simulink model "FuzzyNeuro_neuesNetz"  (Simulink 7.8)
settings: Solver=ode1  StartTime=0.0  StopTime=inf  FixedStep=0.01  RelTol=1e-3
PostLoadFcn:
  | , if any(exist('dsrtsu_mdlpostloadfcn', 'file') == [2, 3, 6]), try dsrtsu_mdlpostloadfcn('Execute', bdroot); catch fprintf('Error in PostLoadFcn (dsrtsu_mdlpostloadfcn) for model "%s":\n %s\n', bdroot, lasterr); end, end,
undefined symbols (not defined in the file): Faktorh1, Faktorh2, Faktorh3, Offseth1, Offseth2, Offseth3
libraries: neural x14, rtilib1104 x13, fuzblock x1
CloseFcn:
  | rtwprivate ssgencode ModelCloseRequest FuzzyNeuro
settings Model: DSRTSU_INTERNAL_RTI_VER=390  DSRTSU_INTERNAL_RTI_TYPE=rti1104  Creator=pendel  LastModifiedBy=pendel  ExtModeArmWhenConnect=off  BufferReuse=off
settings OptimizationCC: BlockReduction=off  BooleanDataType=off  OptimizeBlockIOStorage=off  BufferReuse=off  ExpressionFolding=off  LocalBlockOutputs=off  InitFltsAndDblsToZero=on
settings DebuggingCC: SaveWithParameterizedLinksMsg=none  SignalResolutionControl=TryResolveAllWithWarning  SolverPrmCheckMsg=none  MultiTaskDSMMsg=warning  MultiTaskCondExecSysMsg=none  FcnCallInpInsideContextMsg=Use local settings
settings HardwareCC: ProdIntDivRoundTo=Zero  ProdEndianess=BigEndian  ProdHWDeviceType=Generic->Custom  TargetIntDivRoundTo=Zero  TargetEndianess=BigEndian  TargetHWDeviceType=Generic->Custom
settings RTWCC: SystemTargetFile=rti1104.tlc  MakeCommand=make_rti  TemplateMakefile=rti1104.tmf  Description=dSPACE DS1104 Hardware Platform  RTWVerbose=off  RetainRTWFile=on  ProcessScript=rti1104_make_rtw_hook  IncludeERTFirstTime=on
settings CodeAppCC: IncHierarchyInIds=on
settings STFCustomTargetCC: TargetFcnLib=ansi_tfl_tmw.mat  ParMdlRefBuildCompliant=on  SystemTargetFile=rti1104.tlc
settings GRTTargetCC: TargetFcnLib=ansi_tfl_tmw.mat  CompOptLevelCompliant=off  ConcurrentExecutionCompliant=off  MatFileLogging=off  ExtMode=on  ExtModeMexFile=noextcomm
settings CustomProperty: DataType=RTWOptions_EnumType_C__dSPACE RCPHIL 72_matlab_rti1104_tlc_rti1104_1InitialSimState  Value=RUN
settings EnumStrPairs: String=RUN

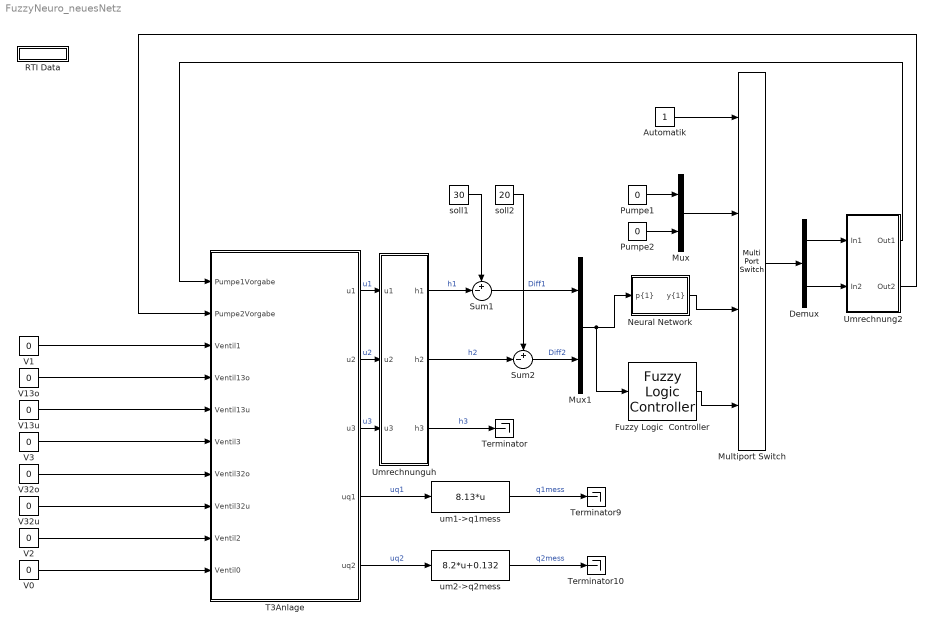
== system FuzzyNeuro_neuesNetz ==
  Automatik : Constant
  Demux : Demux  Outputs=2
  Fuzzy Logic  Controller : fuzblock/Fuzzy Logic  Controller  fis=Schmid
  Multiport Switch : MultiPortSwitch  zeroidx=off  SaturateOnIntegerOverflow=on  InputSameDT=on
  Mux : Mux  Inputs=2
  Mux1 : Mux  Inputs=2
  Neural Network : Subsystem
  Pumpe1 : Constant  Value=0
  Pumpe2 : Constant  Value=0
  RTI Data : Subsystem  Tag=struct('RTIDataServer',struct('RTIDataServerVs','2','RTIModelDescription','struct(''main'',''FuzzyNeuro_neuesNetz'',''sub'','''',''isMp'',0)'))  LoadFcn="if exist('rtidc'), try,  rtidc('DataHostBlockClbLoad', gcbh); catch, disp(['Warning: ''LoadFcn'' for RTI Data block failed: ' lasterr]); end, end,"
      settings: CopyFcn="if exist('rtidc'), try,  rtidc('DataHostBlockClbCopy', gcbh); catch, disp(['Warning: ''CopyFcn'' for RTI Data block failed: ' lasterr]); end, end,"  DeleteFcn="if exist('rtidc'), try,  rtidc('DataHostBlockClbDelete', gcbh); catch, disp(['Warning: ''DeleteFcn'' for RTI Data block failed: ' lasterr]); end, end,"  ModelCloseFcn="if exist('rtidc'), try,  rtidc('DataHostBlockClbModelClose', gcbh); catch, disp(['Warning: ''ModelCloseFcn'' for RTI Data block failed: ' lasterr]); end, end,"  PreSaveFcn="if exist('rtidc'), try,  rtidc('DataHostBlockClbPreSave', gcbh); catch, disp(['Warning: ''PreSaveFcn'' for RTI Data block failed: ' lasterr]); end, end,"  PostSaveFcn="if exist('rtidc'), try,  rtidc('DataHostBlockClbPostSave', gcbh); catch, disp(['Warning: ''PostSaveFcn'' for RTI Data block failed: ' lasterr]); end, end,"  NameChangeFcn="if exist('rtidc'), try,  rtidc('DataHostBlockClbNameChange', gcbh); catch, disp(['Warning: ''NameChangeFcn'' for RTI Data block failed: ' lasterr]); end, end,"
      mask Type: RTI_DATA_HOST
      mask Description:
      | RTI Data Block.
      | This block is used by RTI to store internal model-dependent data.
      | Please keep this block on the root level of the model. Deleting this block will result in data loss.
      | 
      | NEVER DELETE OR COPY THIS BLOCK!
      mask Help:
      | RTI Data Block.
      | This block is used by RTI to store internal model-dependent data.
      | Please keep this block on the root level of the model. Deleting this block will result in data loss.
      | 
      | NEVER DELETE OR COPY THIS BLOCK!
      mask Display:
      | text(0.5, 0.5, 'RTI Data', 'HorizontalAlignment', 'center');
      | plot([1 0]);
  Sum1 : Sum  Inputs=+-|  SaturateOnIntegerOverflow=on  InputSameDT=on  OutDataTypeStr=Inherit: Same as first input
  Sum2 : Sum  Inputs=+-|  SaturateOnIntegerOverflow=on  InputSameDT=on  OutDataTypeStr=Inherit: Same as first input
  T3Anlage : Subsystem
  Terminator : Terminator
  Terminator10 : Terminator
  Terminator9 : Terminator
  Umrechnung2 : Subsystem
  Umrechnunguh : Subsystem
  V{0..3} (4 alike) : Constant  Value=0
  V13o : Constant  Value=0
  V13u : Constant  Value=0
  V32o : Constant  Value=0
  V32u : Constant  Value=0
  soll1 : Constant  Value=30
  soll2 : Constant  Value=20
  um1->q1mess : Fcn  Expr=8.13*u
  um2->q2mess : Fcn  Expr=8.2*u+0.132
  wires:
  Automatik/1 -> Multiport Switch/1
  Multiport Switch/1 -> Demux/1
  T3Anlage/2(u2) -> Umrechnunguh/2(u2)  "u2"
  T3Anlage/3(u3) -> Umrechnunguh/3(u3)  "u3"
  Umrechnunguh/3(h3) -> Terminator/1  "h3"
  Sum2/1 -> Mux1/2  "Diff2"
  soll1/1 -> Sum1/1
  Umrechnunguh/1(h1) -> Sum1/2  "h1"
  Umrechnunguh/2(h2) -> Sum2/2  "h2"
  soll2/1 -> Sum2/1
  Sum1/1 -> Mux1/1  "Diff1"
  Neural Network/1("y{1}") -> Multiport Switch/3
  Mux1/1 -> Fuzzy Logic  Controller/1, Neural Network/1("p{1}")
  Pumpe1/1 -> Mux/1
  Pumpe2/1 -> Mux/2
  Mux/1 -> Multiport Switch/2
  Demux/1 -> Umrechnung2/1(In1)
  Demux/2 -> Umrechnung2/2(In2)
  Umrechnung2/1(Out1) -> T3Anlage/1(Pumpe1Vorgabe)
  Umrechnung2/2(Out2) -> T3Anlage/2(Pumpe2Vorgabe)
  T3Anlage/4(uq1) -> um1->q1mess/1  "uq1"
  um1->q1mess/1 -> Terminator9/1  "q1mess"
  T3Anlage/5(uq2) -> um2->q2mess/1  "uq2"
  um2->q2mess/1 -> Terminator10/1  "q2mess"
  V1/1 -> T3Anlage/3(Ventil1)
  V13o/1 -> T3Anlage/4(Ventil13o)
  V13u/1 -> T3Anlage/5(Ventil13u)
  V3/1 -> T3Anlage/6(Ventil3)
  V32o/1 -> T3Anlage/7(Ventil32o)
  V32u/1 -> T3Anlage/8(Ventil32u)
  V2/1 -> T3Anlage/9(Ventil2)
  V0/1 -> T3Anlage/10(Ventil0)
  T3Anlage/1(u1) -> Umrechnunguh/1(u1)  "u1"
  Fuzzy Logic  Controller/1 -> Multiport Switch/4

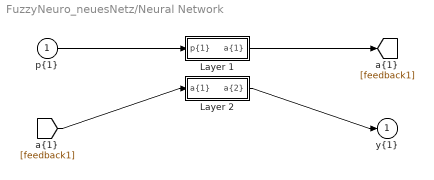
== system FuzzyNeuro_neuesNetz/Neural Network ==
  "p{1}" : Inport  PortDimensions=2  SampleTime=0.01
  Layer 1 : Subsystem
  Layer 2 : Subsystem
  "y{1}" : Outport  InitialOutput=[0;0]
  wires:
  "p{1}"/1 -> Layer 1/1("p{1}")
  Layer 1/1("a{1}") -> [feedback1]
  [feedback1] -> Layer 2/1("a{1} ")
  Layer 2/1("a{2}") -> "y{1}"/1

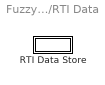
== system FuzzyNeuro_neuesNetz/RTI Data ==
  RTI Data Store : Subsystem  Tag="struct('private',struct('version',struct('dsVer',uint32(2),'dsVerCreation',uint32(2),'RTI',struct('ver','4.2','type','RTI1103')),'access',struct('type','Model','isPerm',1,'created',['14-Aug-2002 15:51:47'],'modified',['05-Nov-2015 18:46:08'],'location','')),'public',struct('main',struct('data',[]),'sub',struct('name',{{'FuzzyNeuro_neuesNetz'}},'data',{{struct('TH',struct('thTaskInfo',struct('taskType',{'TIMER','HWINT','TMRINT','SWINT'},'tasksNumOf',{1,0,0,0},'srcIds',{{'TIMERA'},{},{},{}},'taskNames',{{['Timer Task 1']},{},{},{}})),'th_tc',struct('dataType','TASK','taskGroupId','','taskGroupList',{{}},'taskSchedulingPolicy','FCFS','taskType','TIMER','blkh',-1,'srcId','TIMERA','srcSgnName',['Timer A interrupt'],'srcCpuName','','taskName',['Timer Task 1  [0.01] s'],'taskNameDisplayExt','','smplTime',0.01,'smplTimeOffs',0,'hasFixedPriority',0,'priority',1,'hasFixedOvc',0,'ovcType',1,'ovcMax',0),'tc_th',struct('dataType','TASK','taskGroupId','','taskGroupList',{{}},'taskSchedulingPolicy','FCFS','taskType','TIMER','blkh',-1,'srcId','TIMERA','srcSgnName',['Timer A interrupt'],'srcCpuName','','taskName',['Timer Task 1  [0.01] s'],'taskNameDisplayExt','','smplTime',0.01,'smplTimeOffs',0,'hasFixedPriority',0,'priority',1,'hasFixedOvc',0,'ovcType',1,'ovcMax',0))}})))"
      mask Type: RTI_DATA_STORE
      mask Description:
      | RTI Data Store Block. This block is used by RTI to store internal model dependent data. Deleting this block will result in data loss.
      | 
      | NEVER DELETE, COPY, OR MODIFY THIS BLOCK!
      mask Help:
      | RTI Data Store Block. This block is used by RTI to store internal model dependent data. Deleting this block will result in data loss.
      | 
      | NEVER DELETE, COPY, OR MODIFY THIS BLOCK!
      mask Display: text(0.5, 0.5, ' ', 'HorizontalAlignment', 'center');

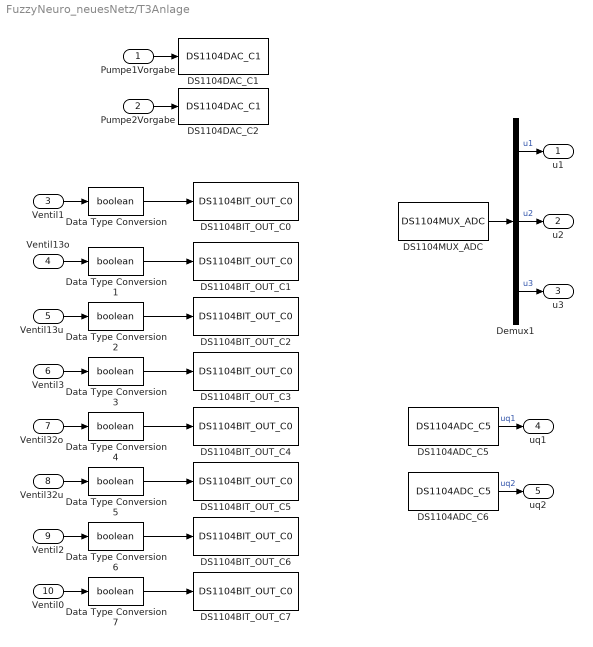
== system FuzzyNeuro_neuesNetz/T3Anlage ==
  Pumpe1Vorgabe : Inport
  Pumpe2Vorgabe : Inport  Port=2
  Ventil1 : Inport  Port=3
  Ventil13o : Inport  Port=4
  Ventil13u : Inport  Port=5
  Ventil3 : Inport  Port=6
  Ventil32o : Inport  Port=7
  Ventil32u : Inport  Port=8
  Ventil2 : Inport  Port=9
  Ventil0 : Inport  Port=10
  DS1104ADC_C5 : rtilib1104/DS1104 MASTER PPC/DS1104ADC_C5  ChannelNo=5  TriggerMode=0  Reserved1=[]  Reserved2=[]  Reserved3=[]  Reserved4=[]  DialogFcn=gui1104adc  UnitName={ 'DS1104ADC_C' }  UnitValues={ 5 }  DSProperties=struct('RTI',struct('Version',uint32(1),'BlockType',struct('isSLSource',uint8(1),'isSLSink',uint8(0),'isHWSource',uint8(1),'isHWSink',uint8(0),'isSetup',uint8(0),'isInline',uint8(1),'isNonInline',uint8(0),'isInterrupt',uint8(0),'isChannelwise',uint8(1)),'IOBoardType','DS1104MASTER','UnitType','ADC','Identifier','ADC','DialogType','ML','BlockSet','NONE','SlaveProcessor','NONE'))
  DS1104ADC_C6 : rtilib1104/DS1104 MASTER PPC/DS1104ADC_C5  ChannelNo=6  TriggerMode=0  Reserved1=[]  Reserved2=[]  Reserved3=[]  Reserved4=[]  DialogFcn=gui1104adc  UnitName={ 'DS1104ADC_C' }  UnitValues={ 6 }  DSProperties=struct('RTI',struct('Version',uint32(1),'BlockType',struct('isSLSource',uint8(1),'isSLSink',uint8(0),'isHWSource',uint8(1),'isHWSink',uint8(0),'isSetup',uint8(0),'isInline',uint8(1),'isNonInline',uint8(0),'isInterrupt',uint8(0),'isChannelwise',uint8(1)),'IOBoardType','DS1104MASTER','UnitType','ADC','Identifier','ADC','DialogType','ML','BlockSet','NONE','SlaveProcessor','NONE'))
  DS1104BIT_OUT_C0 : rtilib1104/DS1104 MASTER PPC/DS1104BIT_OUT_C0  ChannelNo=0  InitValue=0  TermMode=0  TermValue=0  Reserved1=[]  Reserved2=[]  Reserved3=[]  Reserved=[]  DialogFcn=gui1104bit_out  UnitName={'DS1104BIT_OUT_C'}  UnitValues={ 0 }  DSProperties=struct('RTI',struct('Version',uint32(1),'BlockType',struct('isSLSource',uint8(0),'isSLSink',uint8(1),'isHWSource',uint8(0),'isHWSink',uint8(1),'isSetup',uint8(0),'isInline',uint8(1),'isNonInline',uint8(0),'isInterrupt',uint8(0),'isChannelwise',uint8(1)),'IOBoardType','DS1104MASTER','UnitType','BIT','Identifier','BITOUTCH','DialogType','ML','BlockSet','NONE','SlaveProcessor','NONE'))
  DS1104BIT_OUT_C1 : rtilib1104/DS1104 MASTER PPC/DS1104BIT_OUT_C0  ChannelNo=1  InitValue=0  TermMode=0  TermValue=0  Reserved1=[]  Reserved2=[]  Reserved3=[]  Reserved=[]  DialogFcn=gui1104bit_out  UnitName={'DS1104BIT_OUT_C'}  UnitValues={1}  DSProperties=struct('RTI',struct('Version',uint32(1),'BlockType',struct('isSLSource',uint8(0),'isSLSink',uint8(1),'isHWSource',uint8(0),'isHWSink',uint8(1),'isSetup',uint8(0),'isInline',uint8(1),'isNonInline',uint8(0),'isInterrupt',uint8(0),'isChannelwise',uint8(1)),'IOBoardType','DS1104MASTER','UnitType','BIT','Identifier','BITOUTCH','DialogType','ML','BlockSet','NONE','SlaveProcessor','NONE'))
  DS1104BIT_OUT_C2 : rtilib1104/DS1104 MASTER PPC/DS1104BIT_OUT_C0  ChannelNo=2  InitValue=0  TermMode=0  TermValue=0  Reserved1=[]  Reserved2=[]  Reserved3=[]  Reserved=[]  DialogFcn=gui1104bit_out  UnitName={'DS1104BIT_OUT_C'}  UnitValues={2}  DSProperties=struct('RTI',struct('Version',uint32(1),'BlockType',struct('isSLSource',uint8(0),'isSLSink',uint8(1),'isHWSource',uint8(0),'isHWSink',uint8(1),'isSetup',uint8(0),'isInline',uint8(1),'isNonInline',uint8(0),'isInterrupt',uint8(0),'isChannelwise',uint8(1)),'IOBoardType','DS1104MASTER','UnitType','BIT','Identifier','BITOUTCH','DialogType','ML','BlockSet','NONE','SlaveProcessor','NONE'))
  DS1104BIT_OUT_C3 : rtilib1104/DS1104 MASTER PPC/DS1104BIT_OUT_C0  ChannelNo=3  InitValue=0  TermMode=0  TermValue=0  Reserved1=[]  Reserved2=[]  Reserved3=[]  Reserved=[]  DialogFcn=gui1104bit_out  UnitName={'DS1104BIT_OUT_C'}  UnitValues={3}  DSProperties=struct('RTI',struct('Version',uint32(1),'BlockType',struct('isSLSource',uint8(0),'isSLSink',uint8(1),'isHWSource',uint8(0),'isHWSink',uint8(1),'isSetup',uint8(0),'isInline',uint8(1),'isNonInline',uint8(0),'isInterrupt',uint8(0),'isChannelwise',uint8(1)),'IOBoardType','DS1104MASTER','UnitType','BIT','Identifier','BITOUTCH','DialogType','ML','BlockSet','NONE','SlaveProcessor','NONE'))
  DS1104BIT_OUT_C4 : rtilib1104/DS1104 MASTER PPC/DS1104BIT_OUT_C0  ChannelNo=4  InitValue=0  TermMode=0  TermValue=0  Reserved1=[]  Reserved2=[]  Reserved3=[]  Reserved=[]  DialogFcn=gui1104bit_out  UnitName={'DS1104BIT_OUT_C'}  UnitValues={4}  DSProperties=struct('RTI',struct('Version',uint32(1),'BlockType',struct('isSLSource',uint8(0),'isSLSink',uint8(1),'isHWSource',uint8(0),'isHWSink',uint8(1),'isSetup',uint8(0),'isInline',uint8(1),'isNonInline',uint8(0),'isInterrupt',uint8(0),'isChannelwise',uint8(1)),'IOBoardType','DS1104MASTER','UnitType','BIT','Identifier','BITOUTCH','DialogType','ML','BlockSet','NONE','SlaveProcessor','NONE'))
  DS1104BIT_OUT_C5 : rtilib1104/DS1104 MASTER PPC/DS1104BIT_OUT_C0  ChannelNo=5  InitValue=0  TermMode=0  TermValue=0  Reserved1=[]  Reserved2=[]  Reserved3=[]  Reserved=[]  DialogFcn=gui1104bit_out  UnitName={'DS1104BIT_OUT_C'}  UnitValues={5}  DSProperties=struct('RTI',struct('Version',uint32(1),'BlockType',struct('isSLSource',uint8(0),'isSLSink',uint8(1),'isHWSource',uint8(0),'isHWSink',uint8(1),'isSetup',uint8(0),'isInline',uint8(1),'isNonInline',uint8(0),'isInterrupt',uint8(0),'isChannelwise',uint8(1)),'IOBoardType','DS1104MASTER','UnitType','BIT','Identifier','BITOUTCH','DialogType','ML','BlockSet','NONE','SlaveProcessor','NONE'))
  DS1104BIT_OUT_C6 : rtilib1104/DS1104 MASTER PPC/DS1104BIT_OUT_C0  ChannelNo=6  InitValue=0  TermMode=0  TermValue=0  Reserved1=[]  Reserved2=[]  Reserved3=[]  Reserved=[]  DialogFcn=gui1104bit_out  UnitName={'DS1104BIT_OUT_C'}  UnitValues={6}  DSProperties=struct('RTI',struct('Version',uint32(1),'BlockType',struct('isSLSource',uint8(0),'isSLSink',uint8(1),'isHWSource',uint8(0),'isHWSink',uint8(1),'isSetup',uint8(0),'isInline',uint8(1),'isNonInline',uint8(0),'isInterrupt',uint8(0),'isChannelwise',uint8(1)),'IOBoardType','DS1104MASTER','UnitType','BIT','Identifier','BITOUTCH','DialogType','ML','BlockSet','NONE','SlaveProcessor','NONE'))
  DS1104BIT_OUT_C7 : rtilib1104/DS1104 MASTER PPC/DS1104BIT_OUT_C0  ChannelNo=7  InitValue=0  TermMode=0  TermValue=0  Reserved1=[]  Reserved2=[]  Reserved3=[]  Reserved=[]  DialogFcn=gui1104bit_out  UnitName={'DS1104BIT_OUT_C'}  UnitValues={7}  DSProperties=struct('RTI',struct('Version',uint32(1),'BlockType',struct('isSLSource',uint8(0),'isSLSink',uint8(1),'isHWSource',uint8(0),'isHWSink',uint8(1),'isSetup',uint8(0),'isInline',uint8(1),'isNonInline',uint8(0),'isInterrupt',uint8(0),'isChannelwise',uint8(1)),'IOBoardType','DS1104MASTER','UnitType','BIT','Identifier','BITOUTCH','DialogType','ML','BlockSet','NONE','SlaveProcessor','NONE'))
  DS1104DAC_C1 : rtilib1104/DS1104 MASTER PPC/DS1104DAC_C1  ChannelNo=1  InitValue=0  TermMode=0  TermValue=0  Reserved1=[]  Reserved2=[]  Reserved3=[]  Reserved4=[]  DialogFcn=gui1104dac  UnitName={ 'DS1104DAC_C'}  UnitValues={ 1 }  DSProperties=struct('RTI',struct('Version',uint32(1),'BlockType',struct('isSLSource',uint8(0),'isSLSink',uint8(1),'isHWSource',uint8(0),'isHWSink',uint8(1),'isSetup',uint8(0),'isInline',uint8(1),'isNonInline',uint8(0),'isInterrupt',uint8(0),'isChannelwise',uint8(1)),'IOBoardType','DS1104MASTER','UnitType','DAC','Identifier','DAC','DialogType','ML','BlockSet','NONE','SlaveProcessor','NONE'))
  DS1104DAC_C2 : rtilib1104/DS1104 MASTER PPC/DS1104DAC_C1  ChannelNo=2  InitValue=0  TermMode=0  TermValue=0  Reserved1=[]  Reserved2=[]  Reserved3=[]  Reserved4=[]  DialogFcn=gui1104dac  UnitName={ 'DS1104DAC_C'}  UnitValues={2}  DSProperties=struct('RTI',struct('Version',uint32(1),'BlockType',struct('isSLSource',uint8(0),'isSLSink',uint8(1),'isHWSource',uint8(0),'isHWSink',uint8(1),'isSetup',uint8(0),'isInline',uint8(1),'isNonInline',uint8(0),'isInterrupt',uint8(0),'isChannelwise',uint8(1)),'IOBoardType','DS1104MASTER','UnitType','DAC','Identifier','DAC','DialogType','ML','BlockSet','NONE','SlaveProcessor','NONE'))
  DS1104MUX_ADC : rtilib1104/DS1104 MASTER PPC/DS1104MUX_ADC  ChannelNos=[1 2 3]  TriggerMode=0  Reserved1=[]  Reserved2=[]  Reserved3=[]  Reserved4=[]  DialogFcn=gui1104mux_adc  UnitName={ 'DS1104MUX_ADC' }  UnitValues={ [] }  DSProperties=struct('RTI',struct('Version',uint32(1),'BlockType',struct('isSLSource',uint8(1),'isSLSink',uint8(0),'isHWSource',uint8(1),'isHWSink',uint8(0),'isSetup',uint8(0),'isInline',uint8(1),'isNonInline',uint8(0),'isInterrupt',uint8(0),'isChannelwise',uint8(0)),'IOBoardType','DS1104MASTER','UnitType','ADC','Identifier','ADCMUX','DialogType','ML','BlockSet','NONE','SlaveProcessor','NONE'))
  Data Type Conversion{,1..7} (8 alike) : DataTypeConversion  OutDataTypeStr=boolean  SaturateOnIntegerOverflow=on  RndMeth=Zero
  Demux1 : Demux  Outputs=3
  u1 : Outport
  u2 : Outport  Port=2
  u3 : Outport  Port=3
  uq1 : Outport  Port=4
  uq2 : Outport  Port=5
  wires:
  Data Type Conversion/1 -> DS1104BIT_OUT_C0/1
  Data Type Conversion1/1 -> DS1104BIT_OUT_C1/1
  Data Type Conversion2/1 -> DS1104BIT_OUT_C2/1
  Data Type Conversion3/1 -> DS1104BIT_OUT_C3/1
  Data Type Conversion4/1 -> DS1104BIT_OUT_C4/1
  Data Type Conversion5/1 -> DS1104BIT_OUT_C5/1
  Data Type Conversion6/1 -> DS1104BIT_OUT_C6/1
  Data Type Conversion7/1 -> DS1104BIT_OUT_C7/1
  DS1104MUX_ADC/1 -> Demux1/1
  Pumpe1Vorgabe/1 -> DS1104DAC_C1/1
  Pumpe2Vorgabe/1 -> DS1104DAC_C2/1
  Ventil1/1 -> Data Type Conversion/1
  Demux1/1 -> u1/1  "u1"
  Ventil13o/1 -> Data Type Conversion1/1
  Demux1/2 -> u2/1  "u2"
  Ventil13u/1 -> Data Type Conversion2/1
  Ventil3/1 -> Data Type Conversion3/1
  Demux1/3 -> u3/1  "u3"
  Ventil32o/1 -> Data Type Conversion4/1
  Ventil32u/1 -> Data Type Conversion5/1
  DS1104ADC_C5/1 -> uq1/1  "uq1"
  Ventil2/1 -> Data Type Conversion6/1
  DS1104ADC_C6/1 -> uq2/1  "uq2"
  Ventil0/1 -> Data Type Conversion7/1

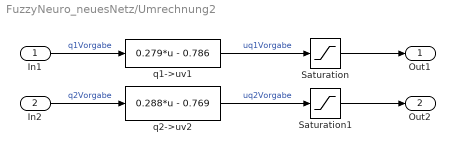
== system FuzzyNeuro_neuesNetz/Umrechnung2 ==
  In1 : Inport
  In2 : Inport  Port=2
  Saturation : Saturate  UpperLimit=1  LowerLimit=-1
  Saturation1 : Saturate  UpperLimit=1  LowerLimit=-1
  q1->uv1 : Fcn  Expr=0.279*u - 0.786
  q2->uv2 : Fcn  Expr=0.288*u - 0.769
  Out1 : Outport  InitialOutput=0
  Out2 : Outport  Port=2  InitialOutput=0
  wires:
  In1/1 -> q1->uv1/1  "q1Vorgabe"
  In2/1 -> q2->uv2/1  "q2Vorgabe"
  q1->uv1/1 -> Saturation/1  "uq1Vorgabe"
  q2->uv2/1 -> Saturation1/1  "uq2Vorgabe"
  Saturation/1 -> Out1/1
  Saturation1/1 -> Out2/1

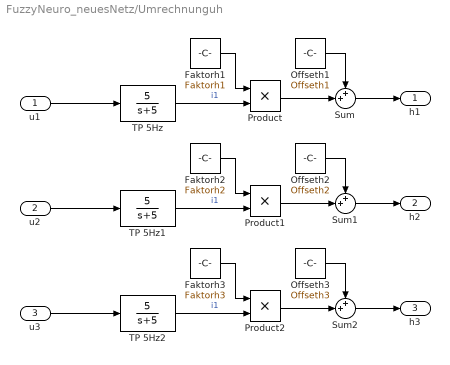
== system FuzzyNeuro_neuesNetz/Umrechnunguh ==
  u1 : Inport
  u2 : Inport  Port=2
  u3 : Inport  Port=3
  Faktorh1 : Constant  Value=Faktorh1
  Faktorh2 : Constant  Value=Faktorh2
  Faktorh3 : Constant  Value=Faktorh3
  Offseth1 : Constant  Value=Offseth1
  Offseth2 : Constant  Value=Offseth2
  Offseth3 : Constant  Value=Offseth3
  Product : Product  SaturateOnIntegerOverflow=on  RndMeth=Zero  InputSameDT=on  OutDataTypeStr=Inherit: Same as first input
  Product1 : Product  SaturateOnIntegerOverflow=on  RndMeth=Zero  InputSameDT=on  OutDataTypeStr=Inherit: Same as first input
  Product2 : Product  SaturateOnIntegerOverflow=on  RndMeth=Zero  InputSameDT=on  OutDataTypeStr=Inherit: Same as first input
  Sum : Sum  Inputs=++|  SaturateOnIntegerOverflow=on  InputSameDT=on  OutDataTypeStr=Inherit: Same as first input
  Sum1 : Sum  Inputs=++|  SaturateOnIntegerOverflow=on  InputSameDT=on  OutDataTypeStr=Inherit: Same as first input
  Sum2 : Sum  Inputs=++|  SaturateOnIntegerOverflow=on  InputSameDT=on  OutDataTypeStr=Inherit: Same as first input
  TP 5Hz : TransferFcn  Numerator=[5]  Denominator=[1 5]
  TP 5Hz1 : TransferFcn  Numerator=[5]  Denominator=[1 5]
  TP 5Hz2 : TransferFcn  Numerator=[5]  Denominator=[1 5]
  h1 : Outport  InitialOutput=0
  h2 : Outport  Port=2  InitialOutput=0
  h3 : Outport  Port=3  InitialOutput=0
  wires:
  Product/1 -> Sum/2
  Sum/1 -> h1/1
  Faktorh1/1 -> Product/1
  Offseth1/1 -> Sum/1
  TP 5Hz/1 -> Product/2  "i1"
  Product2/1 -> Sum2/2
  Sum2/1 -> h3/1
  Faktorh3/1 -> Product2/1
  Offseth3/1 -> Sum2/1
  TP 5Hz2/1 -> Product2/2  "i1"
  Product1/1 -> Sum1/2
  Sum1/1 -> h2/1
  Faktorh2/1 -> Product1/1
  Offseth2/1 -> Sum1/1
  TP 5Hz1/1 -> Product1/2  "i1"
  u2/1 -> TP 5Hz1/1
  u1/1 -> TP 5Hz/1
  u3/1 -> TP 5Hz2/1

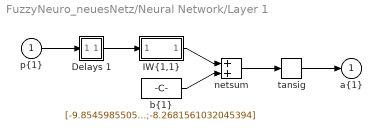
== system FuzzyNeuro_neuesNetz/Neural Network/Layer 1 ==
  "p{1}" : Inport  PortDimensions=2  SampleTime=0.01
  Delays 1 : Subsystem
      mask Display: disp('TDL')
  "IW{1,1}" : Subsystem
      mask Display: disp('weight')
  "b{1}" : Constant  Value=[-9.8545985505022529;3.1869783820136055;-7.8385048556717223;-2.6842174078204861;-1.0793676125527614;-2.1740694877769813;-5.427515514459051;-2.0106026099595997;0.36933408755053759;-8.2681561032045394]
      mask Display: disp('bias')
  netsum : Sum  Inputs=2  SaturateOnIntegerOverflow=on  InputSameDT=on  OutDataTypeStr=Inherit: Same as first input
  tansig : neural/Transfer Functions/tansig
  "a{1}" : Outport  InitialOutput=[0;0;0;0;0;0;0;0;0;0]
  wires:
  "p{1}"/1 -> Delays 1/1("p{1}")
  Delays 1/1("pd{1,1}") -> "IW{1,1}"/1("pd{1,1}")
  "IW{1,1}"/1("iz{1,1}") -> netsum/1
  "b{1}"/1 -> netsum/2
  netsum/1 -> tansig/1
  tansig/1 -> "a{1}"/1

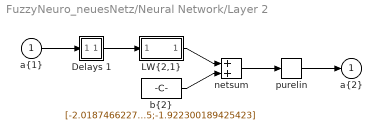
== system FuzzyNeuro_neuesNetz/Neural Network/Layer 2 ==
  "a{1} " : Inport  PortDimensions=10  SampleTime=0.01
  Delays 1 : Subsystem
      mask Display: disp('TDL')
  "LW{2,1}" : Subsystem
      mask Display: disp('weight')
  "b{2}" : Constant  Value=[-2.0187466227910615;-1.922300189425423]
      mask Display: disp('bias')
  netsum : Sum  Inputs=2  SaturateOnIntegerOverflow=on  InputSameDT=on  OutDataTypeStr=Inherit: Same as first input
  purelin : neural/Transfer Functions/purelin
  "a{2}" : Outport  InitialOutput=[0;0]
  wires:
  "a{1} "/1 -> Delays 1/1("p{2}")
  Delays 1/1("pd{2,1}") -> "LW{2,1}"/1("ad{2,1}")
  "LW{2,1}"/1("lz{2,1}") -> netsum/1
  "b{2}"/1 -> netsum/2
  netsum/1 -> purelin/1
  purelin/1 -> "a{2}"/1

== system FuzzyNeuro_neuesNetz/RTI Data/RTI Data Store ==
  RTI Data Store : Subsystem
      mask Type: RTI_DATA_STORE
      mask Description:
      | RTI Data Store Block. This block is used by RTI to store internal model dependent data. Deleting this block will result in data loss.
      | 
      | NEVER DELETE, COPY, OR MODIFY THIS BLOCK!
      mask Help:
      | RTI Data Store Block. This block is used by RTI to store internal model dependent data. Deleting this block will result in data loss.
      | 
      | NEVER DELETE, COPY, OR MODIFY THIS BLOCK!
      mask Display: text(0.5, 0.5, ' ', 'HorizontalAlignment', 'center');

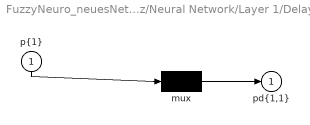
== system FuzzyNeuro_neuesNetz/Neural Network/Layer 1/Delays 1 ==
  "p{1}" : Inport  PortDimensions=2  SampleTime=0.01
  mux : Mux  Inputs=1
  "pd{1,1}" : Outport
  wires:
  "p{1}"/1 -> mux/1
  mux/1 -> "pd{1,1}"/1

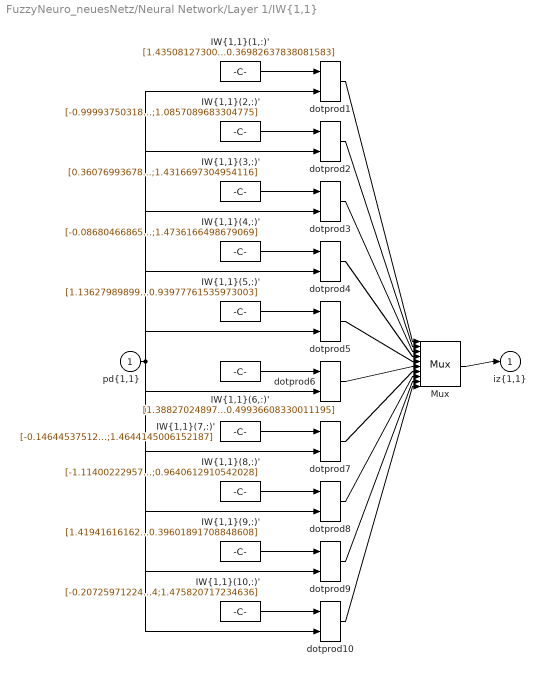
== system FuzzyNeuro_neuesNetz/Neural Network/Layer 1/IW{1,1} ==
  "pd{1,1}" : Inport  PortDimensions=2  SampleTime=0.01
  "IW{1,1}(1,:)'" : Constant  Value=[1.4350812730013165;0.36982637838081583]
      mask Display: disp('weights')
  "IW{1,1}(10,:)'" : Constant  Value=[-0.2072597122421084;1.475820717234636]
      mask Display: disp('weights')
  "IW{1,1}(2,:)'" : Constant  Value=[-0.99993750318269126;1.0857089683304775]
      mask Display: disp('weights')
  "IW{1,1}(3,:)'" : Constant  Value=[0.36076993678749514;1.4316697304954116]
      mask Display: disp('weights')
  "IW{1,1}(4,:)'" : Constant  Value=[-0.086804668652516723;1.4736166498679069]
      mask Display: disp('weights')
  "IW{1,1}(5,:)'" : Constant  Value=[1.1362798989988234;-0.93977761535973003]
      mask Display: disp('weights')
  "IW{1,1}(6,:)'" : Constant  Value=[1.388270248975592;-0.49936608330011195]
      mask Display: disp('weights')
  "IW{1,1}(7,:)'" : Constant  Value=[-0.14644537512169173;1.4644145006152187]
      mask Display: disp('weights')
  "IW{1,1}(8,:)'" : Constant  Value=[-1.1140022295779455;0.9640612910542028]
      mask Display: disp('weights')
  "IW{1,1}(9,:)'" : Constant  Value=[1.4194161616233616;-0.39601891708848608]
      mask Display: disp('weights')
  Mux : Mux  Inputs=10
  dotprod{1..10} (10 alike) : neural/Weight Functions/dotprod
  "iz{1,1}" : Outport
  wires:
  "IW{1,1}(1,:)'"/1 -> dotprod1/1
  "pd{1,1}"/1 -> dotprod1/2, dotprod2/2, dotprod3/2, dotprod4/2, dotprod5/2, dotprod6/2, dotprod7/2, dotprod8/2, dotprod9/2, dotprod10/2
  dotprod1/1 -> Mux/1
  "IW{1,1}(2,:)'"/1 -> dotprod2/1
  dotprod2/1 -> Mux/2
  "IW{1,1}(3,:)'"/1 -> dotprod3/1
  dotprod3/1 -> Mux/3
  "IW{1,1}(4,:)'"/1 -> dotprod4/1
  dotprod4/1 -> Mux/4
  "IW{1,1}(5,:)'"/1 -> dotprod5/1
  dotprod5/1 -> Mux/5
  "IW{1,1}(6,:)'"/1 -> dotprod6/1
  dotprod6/1 -> Mux/6
  "IW{1,1}(7,:)'"/1 -> dotprod7/1
  dotprod7/1 -> Mux/7
  "IW{1,1}(8,:)'"/1 -> dotprod8/1
  dotprod8/1 -> Mux/8
  "IW{1,1}(9,:)'"/1 -> dotprod9/1
  dotprod9/1 -> Mux/9
  "IW{1,1}(10,:)'"/1 -> dotprod10/1
  dotprod10/1 -> Mux/10
  Mux/1 -> "iz{1,1}"/1

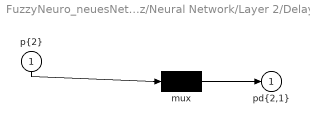
== system FuzzyNeuro_neuesNetz/Neural Network/Layer 2/Delays 1 ==
  "p{2}" : Inport  PortDimensions=10  SampleTime=0.01
  mux : Mux  Inputs=1
  "pd{2,1}" : Outport
  wires:
  "p{2}"/1 -> mux/1
  mux/1 -> "pd{2,1}"/1

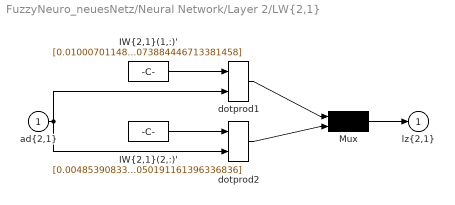
== system FuzzyNeuro_neuesNetz/Neural Network/Layer 2/LW{2,1} ==
  "ad{2,1}" : Inport  PortDimensions=10  SampleTime=0.01
  "IW{2,1}(1,:)'" : Constant  Value=[0.010007011480956507;9.7559540301772607e-005;-0.00045943194759578976;0.00026549758885008323;-0.00037704261757348645;-0.00023329615755329769;-0.0010107765113510359;3.7562430615145637e-005;0.00083885674521977371;0.0073884446713381458]
      mask Display: disp('weights')
  "IW{2,1}(2,:)'" : Constant  Value=[0.0048539083367129532;7.6872455937682105e-005;-0.0013566498908624824;9.8465439347106276e-006;-0.00033394909973916143;6.8337800822604322e-005;0.0018117902613594694;-0.00024838071057661781;0.00040060754880270888;-0.0050191161396336836]
      mask Display: disp('weights')
  Mux : Mux  Inputs=2
  dotprod1 : neural/Weight Functions/dotprod
  dotprod2 : neural/Weight Functions/dotprod
  "lz{2,1}" : Outport
  wires:
  "IW{2,1}(1,:)'"/1 -> dotprod1/1
  "ad{2,1}"/1 -> dotprod1/2, dotprod2/2
  dotprod1/1 -> Mux/1
  "IW{2,1}(2,:)'"/1 -> dotprod2/1
  dotprod2/1 -> Mux/2
  Mux/1 -> "lz{2,1}"/1

== system FuzzyNeuro_neuesNetz/RTI Data/RTI Data Store/RTI Data Store ==
  RTI Data Store : Subsystem
      mask Type: RTI_DATA_STORE
      mask Description:
      | RTI Data Store Block. This block is used by RTI to store internal model dependent data. Deleting this block will result in data loss.
      | 
      | NEVER DELETE, COPY, OR MODIFY THIS BLOCK!
      mask Help:
      | RTI Data Store Block. This block is used by RTI to store internal model dependent data. Deleting this block will result in data loss.
      | 
      | NEVER DELETE, COPY, OR MODIFY THIS BLOCK!
      mask Display: text(0.5, 0.5, ' ', 'HorizontalAlignment', 'center');

== system FuzzyNeuro_neuesNetz/RTI Data/RTI Data Store/RTI Data Store/RTI Data Store ==
  RTI Data Store : Subsystem
      mask Type: RTI_DATA_STORE
      mask Description:
      | RTI Data Store Block. This block is used by RTI to store internal model dependent data. Deleting this block will result in data loss.
      | 
      | NEVER DELETE, COPY, OR MODIFY THIS BLOCK!
      mask Help:
      | RTI Data Store Block. This block is used by RTI to store internal model dependent data. Deleting this block will result in data loss.
      | 
      | NEVER DELETE, COPY, OR MODIFY THIS BLOCK!
      mask Display: text(0.5, 0.5, ' ', 'HorizontalAlignment', 'center');

== system FuzzyNeuro_neuesNetz/RTI Data/RTI Data Store/RTI Data Store/RTI Data Store/RTI Data Store ==
